simulink model "model_advanced_2_pulley"  (R2023b)
settings: Solver=VariableStepAuto  StartTime=0.0  StopTime=t_time  RelTol=1e-3
undefined symbols (not defined in the file or in its folder): const_rot
libraries: sdl_lib x4, fl_lib x3, nesl_utility x2
settings Model: Creator=enrico  LastModifiedBy=enrico
settings DataIOCC: SaveOutput=off  DSMLogging=off  SaveTime=off  ReturnWorkspaceOutputs=off
settings SimscapeCC: SimscapeLogType=all  SimscapeLogSimulationStatistics=on  SimscapeLogToSDI=on

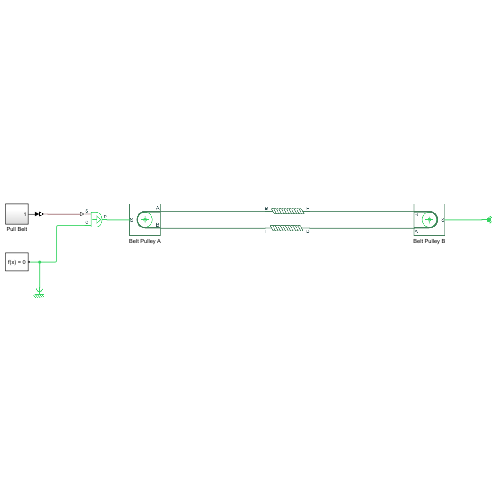
[thumbnail: Simulink's stored preview of the top-level diagram]
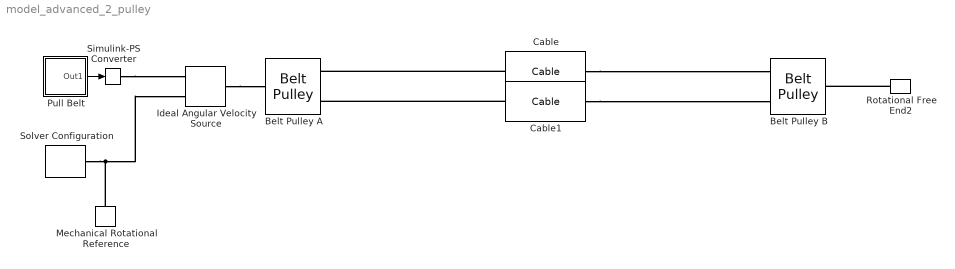
== system model_advanced_2_pulley ==
  Belt Pulley A : sdl_lib/Couplings & Drives/Belt Pulley  belt_type=sdl.enum.belt_type.ideal  sheave_ang=30 deg  num_belts=1  model_f_c=sdl.enum.model_centrifugal.off  linear_density=0.6 kg/m  belt_direction=sdl.enum.belt_direction.opposite  breakable=sdl.enum.max_tension.off  F_max=1e5 N  check_tension=sdl.enum.tension_check.off  pulley_moveable=simscape.enum.onoff.off  r_pulley=radiusA m  b_pulley=0.001 N*m*s/rad  model_inertia=sdl.enum.model_inertia.off  pulley_mass=0.01 kg  initial_vel=0 m/s  pulley_inertia=0.001 kg*m^2  initial_velocity=0 rad/s  friction_model=sdl.enum.PulleyModel.Modal  initial_state_locked=sdl.enum.initial_lock.unlocked  mu=0.5  mu_static=0.5  mu_kinetic=0.42  phi_wrap=180 deg  v_thr=0.001 m/s  f_thr=0.01 N
      settings: InternalSimscapePortConfiguration="{\"Bottom\":[],\"Left\":[{\"id\":\"S\",\"label\":\"S\",\"type\":\"foundation.mechanical.rotational.rotational\"}],\"Right\":[{\"id\":\"A\",\"label\":\"A\",\"type\":\"foundation.mechanical.translational.translational\"},{\"id\":\"B\",\"label\":\"B\",\"type\":\"foundation.mechanical.translational.translational\"}],\"Top\":[]}"
  Belt Pulley B : sdl_lib/Couplings & Drives/Belt Pulley  belt_type=sdl.enum.belt_type.ideal  sheave_ang=30 deg  num_belts=1  model_f_c=sdl.enum.model_centrifugal.off  linear_density=0.6 kg/m  belt_direction=sdl.enum.belt_direction.opposite  breakable=sdl.enum.max_tension.off  F_max=1e5 N  check_tension=sdl.enum.tension_check.off  pulley_moveable=simscape.enum.onoff.off  r_pulley=radiusB m  b_pulley=0.001 N*m*s/rad  model_inertia=sdl.enum.model_inertia.off  pulley_mass=0.01 kg  initial_vel=0 m/s  pulley_inertia=0.01 kg*m^2  initial_velocity=0 rad/s  friction_model=sdl.enum.PulleyModel.Modal  initial_state_locked=sdl.enum.initial_lock.unlocked  mu=0.5  mu_static=0.5  mu_kinetic=0.42  phi_wrap=180 deg  v_thr=0.001 m/s  f_thr=0.01 N
      settings: LogSimulationData=on  InternalSimscapePortConfiguration="{\"Bottom\":[],\"Left\":[{\"id\":\"S\",\"label\":\"S\",\"type\":\"foundation.mechanical.rotational.rotational\"}],\"Right\":[{\"id\":\"A\",\"label\":\"A\",\"type\":\"foundation.mechanical.translational.translational\"},{\"id\":\"B\",\"label\":\"B\",\"type\":\"foundation.mechanical.translational.translational\"}],\"Top\":[]}"
  Cable : sdl_lib/Couplings & Drives/Cable  model_slack=false  cable_parameterization=sdl.enum.ConstantTLU.Constant  model_mass=false  mass=1 kg  stiffness=stiffness N/m  damping=damping N*s/m  stretch_vector=[.1, .2, .5, 1] m  stiffness_vector=[500, 600, 800, 1000] N/m  damping_vector=[50, 60, 80, 100] N*s/m  slack_model=sdl.enum.SlackBoundary.smooth  transition=0.1 mm  breakable=false  f_max=1e5 N  check_tension=false  s_specify=off  s_priority=High  s=0.01 m  s_nominal_specify=off  s_nominal_unit=m  s_nominal_value=1  v_specify=off  v_priority=None  v=0 m/s  v_nominal_specify=off  v_nominal_unit=m/s  v_nominal_value=1  f_specify=off  f_priority=None  f=10 N  f_nominal_specify=on  f_nominal_unit=N  f_nominal_value=1
      settings: InternalSimscapePortConfiguration="{\"Bottom\":[],\"Left\":[{\"id\":\"B\",\"label\":\"B\",\"type\":\"foundation.mechanical.translational.translational\"}],\"Right\":[{\"id\":\"F\",\"label\":\"F\",\"type\":\"foundation.mechanical.translational.translational\"}],\"Top\":[]}"
  Cable1 : sdl_lib/Couplings & Drives/Cable  model_slack=false  cable_parameterization=sdl.enum.ConstantTLU.Constant  model_mass=false  mass=1 kg  stiffness=stiffness N/m  damping=damping N*s/m  stretch_vector=[.1, .2, .5, 1] m  stiffness_vector=[500, 600, 800, 1000] N/m  damping_vector=[50, 60, 80, 100] N*s/m  slack_model=sdl.enum.SlackBoundary.smooth  transition=0.1 mm  breakable=false  f_max=1e5 N  check_tension=false  s_specify=off  s_priority=High  s=0.01 m  s_nominal_specify=off  s_nominal_unit=m  s_nominal_value=1  v_specify=off  v_priority=None  v=0 m/s  v_nominal_specify=off  v_nominal_unit=m/s  v_nominal_value=1  f_specify=off  f_priority=None  f=10 N  f_nominal_specify=on  f_nominal_unit=N  f_nominal_value=1
      settings: InternalSimscapePortConfiguration="{\"Bottom\":[],\"Left\":[{\"id\":\"B\",\"label\":\"B\",\"type\":\"foundation.mechanical.translational.translational\"}],\"Right\":[{\"id\":\"F\",\"label\":\"F\",\"type\":\"foundation.mechanical.translational.translational\"}],\"Top\":[]}"
  Ideal Angular Velocity Source : fl_lib/Mechanical/Mechanical Sources/Ideal Angular Velocity Source
  Mechanical Rotational Reference : fl_lib/Mechanical/Rotational Elements/Mechanical Rotational Reference
  Pull Belt : Subsystem
  Rotational Free End2 : fl_lib/Mechanical/Rotational Elements/Rotational Free End  w_specify=off  w_priority=None  w=0 rad/s  w_nominal_specify=off  w_nominal_unit=rad/s  w_nominal_value=1
  Simulink-PS Converter : nesl_utility/Simulink-PS Converter  PhysicalDomain=network_engine_domain  SubClassName=ps_input  LeftPortType=input  RightPortType=output  PseudoPeriodic=off  Frequencies=[]  NoiseDistribution=none  NoiseParameters=[]  Unit=1  AffineConversion=off  FilteringAndDerivatives=provide  SimscapeFilterOrder=1  InputFilterTimeConstant=0.001  UdotUserProvided=0
  Solver Configuration : nesl_utility/Solver Configuration  PhysicalDomain=network_engine_domain  SubClassName=solver  LeftPortType=input  RightPortType=generic  Tones=[]  Harmonics=[]  SimulateNoise=off  Profile=off  UseLocalSampling=off  EnableSwitchedLinearOptims=on  FrequencyDomain=off  UseCCode=off  RelTol=0.001  AbsTol=1e-06  MinStep=1e-09  ToWorkspace=off  RevertToSquareIcSolve=off  NumHomotopyIterations=100  PhasorMode=off  PhasorModeNumHarmonics=1  ConsistencySolver=NEWTON_FTOL  IndexReductionMethod=DerivativeReplacement  DoDC=off  ResidualTolerance=1e-09  ConsistencyTolSource=GLOBAL  ConsistencyAbsTol=0.001  ConsistencyRelTol=0.001  ConsistencyTolFactor=0.001  UseLocalSolver=off  LocalSolverChoice=NE_BACKWARD_EULER_ADVANCER  ResolveIndetEquations=on  FunctionEvalNumThread=1  LocalSolverSampleTime=0.001  DoFixedCost=off  MaxNonlinIter=3  MaxModeIter=2  ComputeImpulses=off  ImpulseIterations=1  LinearAlgebra=Sparse  LinearAlgebraNumThread=0  EquationFormulation=NE_TIME_EF  DelaysMemoryBudget=1024  AutomaticFiltering=on  FilteringTimeConstant=0.001  PartitionStorageMethod=AS_NEEDED  PartitionMemoryBudget=1024  PartitionMethod=FAST  MultibodyUseLocalSolver=off  MultibodyLocalSolverChoice=ODE1  MultibodyLocalSolverSampleTime=0.001
  wires:
  Pull Belt/1(Out1) -> Simulink-PS Converter/1
  connections:
  Mechanical Rotational Reference/LConn1 -- Ideal Angular Velocity Source/RConn2 -- Solver Configuration/RConn1
  Ideal Angular Velocity Source/LConn1 -- Belt Pulley A/LConn1
  Simulink-PS Converter/RConn1 -- Ideal Angular Velocity Source/RConn1
  Rotational Free End2/LConn1 -- Belt Pulley B/LConn1
  Cable/RConn1 -- Belt Pulley B/RConn2
  Cable/LConn1 -- Belt Pulley A/RConn1
  Cable1/LConn1 -- Belt Pulley B/RConn1
  Cable1/RConn1 -- Belt Pulley A/RConn2

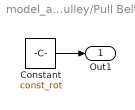
== system model_advanced_2_pulley/Pull Belt ==
  Constant : Constant  Value=const_rot
  Out1 : Outport
  wires:
  Constant/1 -> Out1/1
